simulink model "AC"  (R2024b)
settings: Solver=VariableStepAuto  StartTime=0.0  StopTime=inf  RelTol=1e-3
settings Model: PacingRate=0.110000  Creator=HP  LastModifiedBy=HP

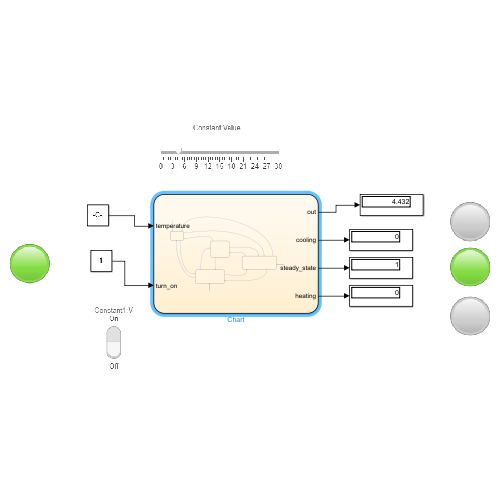
[thumbnail: Simulink's stored preview of the top-level diagram]
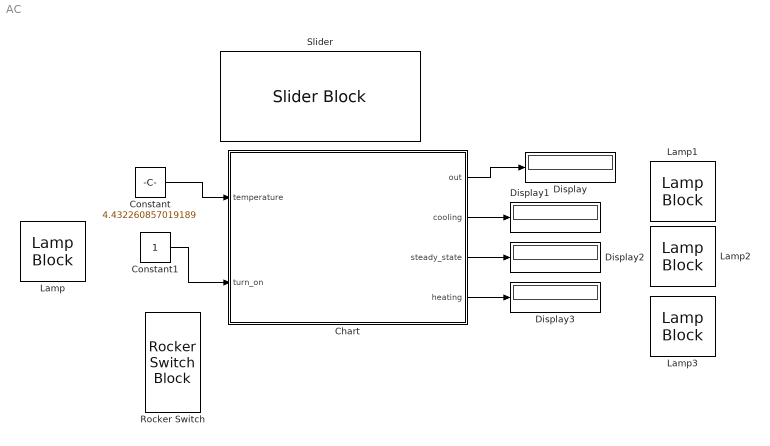
== system AC ==
  Chart : Stateflow chart  TreatAsAtomicUnit=on
  Constant : Constant  Value=4.432260857019189
  Constant1 : Constant
  Display{,1..3} (4 alike) : Display
  Lamp{,1..3} (4 alike) : LampBlock  LabelPosition=Hide
  Rocker Switch : RockerSwitchBlock
      settings: Values={{'Off', 'On'}, [0 1]}
  Slider : SliderBlock  ScaleMax=30
  wires:
  Chart/1(out) -> Display/1
  Constant/1 -> Chart/1(temperature)
  Constant1/1 -> Chart/2(turn_on)
  Chart/2(cooling) -> Display1/1
  Chart/3(steady_state) -> Display2/1
  Chart/4(heating) -> Display3/1

== stateflow chart AC/Chart ==
  state on_off
    out=0
  state steady
    entry:
    steady_state=1;
    out=heat_temp;
    exit:
    steady_state=0;
  state heat_on
    entry:heating=1;
    heat_temp=heat_temp+(temperature-...
    heat_temp);
    out=heat_temp;
    exit:heating=0;
  state cooler_on
    entry:cooling=1;
    heat_temp=heat_temp-...
    (heat_temp- temperature);
    out=heat_temp;
    exit:cooling=0
  heat_on -> on_off [order 4] : [turn_on==0]
  (default) -> on_off : {heat_temp=0}
  on_off -> heat_on [order 1] : [turn_on==1&&heat_temp<temperature]
  steady -> on_off [order 1] : [turn_on==0]
  cooler_on -> on_off [order 4] : [turn_on==0]
  on_off -> cooler_on [order 2] : [turn_on==1&&heat_temp>temperature]
  steady -> heat_on [order 2] : [turn_on==1&&heat_temp<temperature]
  cooler_on -> steady [order 1] : [heat_temp==temperature]
  heat_on -> steady [order 2] : [heat_temp==temperature]
  steady -> cooler_on [order 3] : [turn_on==1&&heat_temp>temperature]
  heat_on -> heat_on [order 3] : [heat_temp<temperature]
  heat_on -> cooler_on [order 1] : [heat_temp>temperature]
  cooler_on -> heat_on [order 2] : [heat_temp<temperature]
  cooler_on -> cooler_on [order 3] : [heat_temp>temperature]
  data: temperature input; turn_on input; out output; heat_temp local; cooling output; steady_state output; heating output
